simulink model "MiniHR"  (R2023a)
settings: Solver=FixedStepAuto  StartTime=0.0  StopTime=90  RelTol=1e-3
PreLoadFcn:
  | k=0.0001;
InitFcn:
  | k=0.0001;
values from neighbouring files (symbols this model uses):
  X = T(4)    [arm_contr.m]
  Y = T(5)    [arm_contr.m]
  Z = T(6)    [arm_contr.m]
libraries: sm_lib x208, nesl_utility x28, simulink x2
(part 2 of 6)

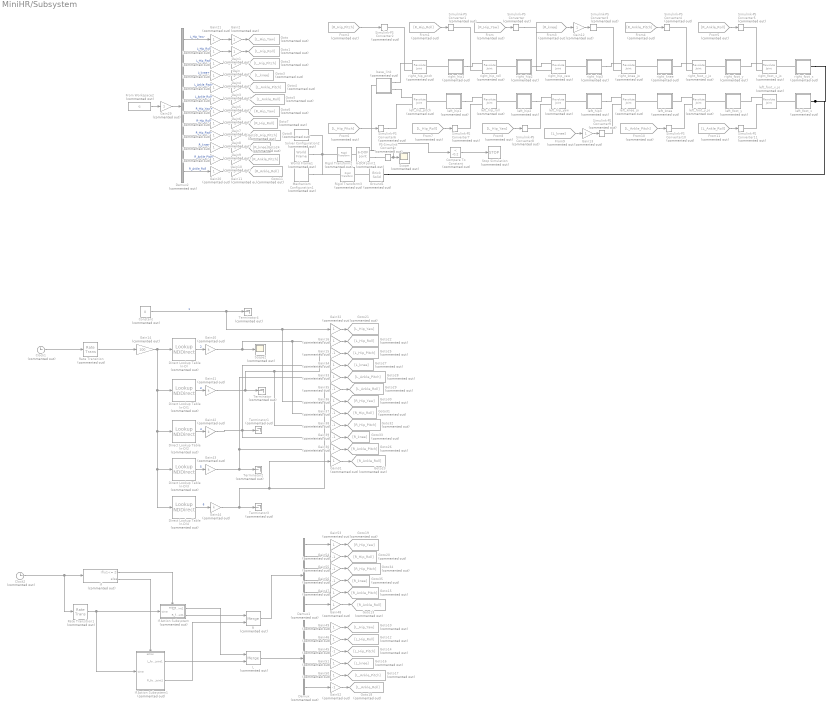
== system MiniHR/Subsystem ==
  6-DOF Joint1 : sm_lib/Joints/6-DOF Joint  Commented=on  JointMode=Normal  SenseConstraintForce=off  SenseConstraintForceX=off  SenseConstraintForceY=off  SenseConstraintForceZ=off  SenseConstraintTorque=off  SenseConstraintTorqueX=off  SenseConstraintTorqueY=off  SenseConstraintTorqueZ=off  SenseTotalForce=off  SenseTotalForceX=off  SenseTotalForceY=off  SenseTotalForceZ=off  SenseTotalTorque=off  SenseTotalTorqueX=off  SenseTotalTorqueY=off  SenseTotalTorqueZ=off  CompositeWrenchDir=FollowerOnBase  CompositeWrenchFrame=BaseFrame  PxEquilibriumPosition=0  PxEquilibriumPositionUnits=m  PxSpringStiffness=0  PxSpringStiffnessUnits=N/m  PxDampingCoefficient=0  PxDampingCoefficientUnits=N/(m/s)  PxTorqueActuationMode=NoTorque  PxMotionActuationMode=ComputedMotion  PxSensePosition=off  PxSenseVelocity=off  PxSenseAcceleration=off  PxSenseTorqueForce=off  PxSenseLowerLimitTorqueForce=off  PxSenseUpperLimitTorqueForce=off  PxLowerLimitSpecify=off  PxLowerLimitBound=-1  PxLowerLimitBoundUnits=m  PxLowerLimitStiffness=1e6  PxLowerLimitStiffnessUnits=N/m  PxLowerLimitDamping=1e3  PxLowerLimitDampingUnits=N/(m/s)  PxLowerLimitTransitionRegionWidth=1e-4  PxLowerLimitTransitionRegionWidthUnits=m  PxUpperLimitSpecify=off  PxUpperLimitBound=1  PxUpperLimitBoundUnits=m  PxUpperLimitStiffness=1e6  PxUpperLimitStiffnessUnits=N/m  PxUpperLimitDamping=1e3  PxUpperLimitDampingUnits=N/(m/s)  PxUpperLimitTransitionRegionWidth=1e-4  PxUpperLimitTransitionRegionWidthUnits=m  PxPositionTargetSpecify=off  PxPositionTargetPriority=High  PxPositionTargetValue=0  PxPositionTargetValueUnits=m  PxVelocityTargetSpecify=off  PxVelocityTargetPriority=High  PxVelocityTargetValue=0  PxVelocityTargetValueUnits=m/s  PyEquilibriumPosition=0  PyEquilibriumPositionUnits=m  PySpringStiffness=0  PySpringStiffnessUnits=N/m  PyDampingCoefficient=0  PyDampingCoefficientUnits=N/(m/s)  PyTorqueActuationMode=NoTorque  PyMotionActuationMode=ComputedMotion  PySensePosition=off  PySenseVelocity=off  PySenseAcceleration=off  PySenseTorqueForce=off  PySenseLowerLimitTorqueForce=off  PySenseUpperLimitTorqueForce=off  PyLowerLimitSpecify=off  PyLowerLimitBound=-1  PyLowerLimitBoundUnits=m  PyLowerLimitStiffness=1e6  PyLowerLimitStiffnessUnits=N/m  PyLowerLimitDamping=1e3  PyLowerLimitDampingUnits=N/(m/s)  PyLowerLimitTransitionRegionWidth=1e-4  PyLowerLimitTransitionRegionWidthUnits=m  PyUpperLimitSpecify=off  PyUpperLimitBound=1  PyUpperLimitBoundUnits=m  PyUpperLimitStiffness=1e6  PyUpperLimitStiffnessUnits=N/m  PyUpperLimitDamping=1e3  PyUpperLimitDampingUnits=N/(m/s)  PyUpperLimitTransitionRegionWidth=1e-4  PyUpperLimitTransitionRegionWidthUnits=m  PyPositionTargetSpecify=off  PyPositionTargetPriority=High  PyPositionTargetValue=0  PyPositionTargetValueUnits=m  PyVelocityTargetSpecify=off  PyVelocityTargetPriority=High  PyVelocityTargetValue=0  PyVelocityTargetValueUnits=m/s  PzEquilibriumPosition=0  PzEquilibriumPositionUnits=m  PzSpringStiffness=0  PzSpringStiffnessUnits=N/m  PzDampingCoefficient=0  PzDampingCoefficientUnits=N/(m/s)  PzTorqueActuationMode=NoTorque  PzMotionActuationMode=ComputedMotion  PzSensePosition=on  PzSenseVelocity=off  PzSenseAcceleration=off  PzSenseTorqueForce=off  PzSenseLowerLimitTorqueForce=off  PzSenseUpperLimitTorqueForce=off  PzLowerLimitSpecify=off  PzLowerLimitBound=-1  PzLowerLimitBoundUnits=m  PzLowerLimitStiffness=1e6  PzLowerLimitStiffnessUnits=N/m  PzLowerLimitDamping=1e3  PzLowerLimitDampingUnits=N/(m/s)  PzLowerLimitTransitionRegionWidth=1e-4  PzLowerLimitTransitionRegionWidthUnits=m  PzUpperLimitSpecify=off  PzUpperLimitBound=1  PzUpperLimitBoundUnits=m  PzUpperLimitStiffness=1e6  PzUpperLimitStiffnessUnits=N/m  PzUpperLimitDamping=1e3  PzUpperLimitDampingUnits=N/(m/s)  PzUpperLimitTransitionRegionWidth=1e-4  PzUpperLimitTransitionRegionWidthUnits=m  PzPositionTargetSpecify=off  PzPositionTargetPriority=High  PzPositionTargetValue=0  PzPositionTargetValueUnits=m  PzVelocityTargetSpecify=off  PzVelocityTargetPriority=High  PzVelocityTargetValue=0  PzVelocityTargetValueUnits=m/s  SphEqPosRotationMethod=None  SphEqPosRotationAngleUnits=deg  SphEqPosRotationStandardAxis=+Z  SphEqPosRotationAngle=0.0  SphEqPosRotationArbitraryAxis=[0 0 1]  SphEqPosFollAlignAxisA=+X  SphEqPosBaseAlignAxisA=+Y  SphEqPosFollAlignAxisB=+Y  SphEqPosBaseAlignAxisB=+Z  SphEqPosRotationSequenceAxes=FollowerAxes  SphEqPosRotationSequence=XYX  SphEqPosRotationSequenceAngles=[0 0 0]  SphEqPosRotationSequenceAnglesUnits=deg  SphEqPosRotationMatrix=[1 0 0; 0 1 0; 0 0 1]  SphEqPosQuaternion=[1 0 0 0]  SphSpringStiffness=0  SphSpringStiffnessUnits=N*m/deg  SphDampingCoefficient=0  SphDampingCoefficientUnits=N*m/(deg/s)  SphActuateTorqueX=off  SphActuateTorqueY=off  SphActuateTorqueZ=off  SphActuateTorque=off  SphTorqueActuationMode=NoTorque  SphMotionActuationMode=ComputedMotion  SphActuationFrame=BaseFrame  SphSensePosition=off  SphSenseVelocityX=off  SphSenseVelocityY=off  SphSenseVelocityZ=off  SphSenseVelocity=off  SphSenseAccelerationX=off  SphSenseAccelerationY=off  SphSenseAccelerationZ=off  SphSenseAcceleration=off  SphSenseTorqueX=off  SphSenseTorqueY=off  SphSenseTorqueZ=off  SphSenseTorqueForce=off  SphSenseLowerLimitTorqueMag=off  SphSenseUpperLimitTorqueMag=off  SphSensingFrame=BaseFrame  SphLowerLimitSpecify=off  SphLowerLimitBound=15  SphLowerLimitBoundUnits=deg  SphLowerLimitStiffness=1e4  SphLowerLimitStiffnessUnits=N*m/deg  SphLowerLimitDamping=10  SphLowerLimitDampingUnits=N*m/(deg/s)  SphLowerLimitTransitionRegionWidth=0.1  SphLowerLimitTransitionRegionWidthUnits=deg  SphUpperLimitSpecify=off  SphUpperLimitBound=45  SphUpperLimitBoundUnits=deg  SphUpperLimitStiffness=1e4  SphUpperLimitStiffnessUnits=N*m/deg  SphUpperLimitDamping=10  SphUpperLimitDampingUnits=N*m/(deg/s)  SphUpperLimitTransitionRegionWidth=0.1  SphUpperLimitTransitionRegionWidthUnits=deg  SphPositionTargetRotationMethod=None  SphPositionTargetRotationAngleUnits=deg  SphPositionTargetRotationStandardAxis=+Z  SphPositionTargetRotationAngle=0.0  SphPositionTargetRotationArbitraryAxis=[0 0 1]  SphPositionTargetFollAlignAxisA=+X  SphPositionTargetBaseAlignAxisA=+Y  SphPositionTargetFollAlignAxisB=+Y  SphPositionTargetBaseAlignAxisB=+Z  SphPositionTargetRotationSequenceAxes=FollowerAxes  SphPositionTargetRotationSequence=XYX  SphPositionTargetRotationSequenceAngles=[0 0 0]  SphPositionTargetRotationSequenceAnglesUnits=deg  SphPositionTargetRotationMatrix=[1 0 0; 0 1 0; 0 0 1]  SphPositionTargetQuaternion=[1 0 0 0]  SphPositionTargetSpecify=off  SphPositionTargetPriority=High  SphVelocityTargetValue=[0 0 0]  SphVelocityTargetValueUnits=deg/s  SphVelocityTargetSpecify=off  SphVelocityTargetPriority=High  SphVelocityTargetInFollowerFrame=on
  Clock1 : Clock  Commented=on
  Clock2 : Clock  Commented=on
      settings: Decimation=5
  Compare To Constant : simulink/Logic and Bit Operations/Compare To Constant  Commented=on  relop=<  const=-0.2  OutDataTypeStr=boolean
  Constant : Constant  Commented=on  Value=0  SampleTime=0.01
  Demux : Demux  Commented=on  Outputs=6
  Demux1 : Demux  Commented=on  Outputs=6
  Demux2 : Demux  Commented=on  Outputs=12
  Direct Lookup Table (n-D) : LookupNDDirect  Commented=on  NumberOfTableDimensions=1  Table=[0;0;0;0;0;0;0;0;0;0;0;0;0;0;0;0;0;0;0;0;0;0;0;0;0;0;0;0;0;0;0;0;0;0;0;0;0;0;0;0;0;0;0;0;0;0;0;0;0;0;0;0;0;0;0;0;0;0;0;0;0;0;0;0;0;0;0;0;0;0;0;0;0;0;0;0;0;0;0;0;0;0;0;0;0;0;0;0;0;0;0;0;0;0;0;0;0;0;0;0;0;0;0;0;0;-1;-1;-2;-4;-6;-9;-12;-17;-22;-29;-37;-46;-57;-69;-83;-99;-117;-137;-159;-183;-209;-238;-269;-303;-339;-378;-420;-463;-510;-559;-610;-664;-720;-779;-839;-902;-966;-1032;-1100;-1169;-1238;-1309;-1380;-1451;-1523;-1593;-1664;-1733;-1802;-1873;-1945;-2018;-2091;-2165;-2238;-2311;-2382;-2452;-2519;-2584;-2644;-2700;-2751;-2795;-2832;-2861;-2882;-2892;-2892;-2881;-2857;-2824;-2781;-2725;-2658;-2580;-2493;-2397;-2294;-2183;-2067;-1946;-1821;-1693;-1562;-1428;-1293;-1157;-1020;-882;-744;-605;-466;-327;-187;-47]  RemoveProtectionInput=on
  Direct Lookup Table (n-D)1 : LookupNDDirect  Commented=on  NumberOfTableDimensions=1  Table=[0;0;0;0;0;0;0;0;0;0;0;0;0;0;0;0;0;0;0;0;0;0;0;0;0;0;0;0;0;0;0;0;0;0;0;0;0;0;0;0;0;0;0;0;0;0;0;0;0;0;223;277;396;536;683;832;981;1128;1274;1418;1560;1699;1837;1971;2103;2233;2360;2484;2606;2724;2840;2953;3063;3170;3273;3374;3472;3566;3657;3745;3830;3911;3989;4063;4134;4201;4264;4324;4380;4432;4480;4524;4564;4600;4631;4658;4681;4698;4711;4719;4719;4719;4719;4719;4719;4719;4719;4719;4719;4719;4719;4719;4719;4719;4719;4719;4719;4719;4719;4719;4718;4718;4718;4717;4717;4716;4716;4715;4713;4712;4710;4708;4706;4703;4700;4696;4692;4687;4682;4676;4669;4662;4654;4645;4635;4624;4613;4601;4588;4574;4560;4545;4530;4524;4538;4568;4614;4671;4739;4816;4898;4984;5072;5161;5249;5335;5418;5495;5567;5633;5692;5742;5783;5815;5835;5845;5848;5846;5830;5803;5766;5719;5663;5599;5529;5452;5372;5287;5201;5114;5029;4946;4869;4799;4738;4689;4655;4637;4638;4648;4655]  RemoveProtectionInput=on
  Direct Lookup Table (n-D)2 : LookupNDDirect  Commented=on  NumberOfTableDimensions=1  Table=[0;0;0;0;0;0;0;0;0;0;0;0;0;0;0;0;0;0;0;0;0;0;0;0;0;0;0;0;0;0;0;0;0;0;0;0;0;0;0;0;0;0;0;0;0;0;0;0;0;0;552;688;983;1332;1697;2067;2437;2805;3169;3528;3883;4233;4578;4917;5250;5577;5899;6214;6523;6826;7123;7412;7695;7972;8241;8503;8758;9005;9244;9476;9700;9916;10123;10322;10511;10692;10864;11026;11178;11320;11452;11573;11683;11781;11868;11943;12005;12054;12090;12112;12112;12112;12112;12112;12112;12112;12112;12112;12112;12112;12112;12112;12112;12112;12112;12112;12112;12112;12111;12111;12110;12110;12109;12108;12106;12105;12103;12100;12097;12093;12088;12082;12076;12068;12059;12049;12037;12024;12009;11992;11974;11953;11930;11905;11878;11849;11817;11784;11748;11711;11671;11631;11588;11573;11611;11694;11819;11980;12169;12382;12614;12858;13110;13366;13622;13873;14117;14349;14566;14766;14944;15100;15228;15326;15392;15420;15432;15424;15376;15291;15174;15028;14856;14662;14449;14221;13981;13733;13482;13231;12986;12751;12532;12335;12165;12029;11933;11884;11887;11914;11934]  RemoveProtectionInput=on
  Direct Lookup Table (n-D)3 : LookupNDDirect  Commented=on  NumberOfTableDimensions=1  Table=[0;0;0;0;0;0;0;0;0;0;0;0;0;0;0;0;0;0;0;0;0;0;0;0;0;0;0;0;0;0;0;0;0;0;0;0;0;0;0;0;0;0;0;0;0;0;0;0;0;0;330;411;587;795;1014;1235;1456;1676;1895;2110;2323;2534;2741;2945;3146;3344;3539;3730;3918;4102;4283;4460;4633;4802;4967;5129;5286;5439;5587;5731;5870;6005;6134;6259;6378;6491;6599;6702;6798;6888;6972;7048;7119;7181;7237;7285;7324;7356;7379;7393;7393;7393;7393;7393;7393;7393;7393;7393;7393;7393;7393;7393;7393;7393;7393;7393;7393;7393;7393;7392;7392;7392;7391;7390;7389;7388;7387;7385;7383;7381;7378;7374;7370;7365;7359;7353;7345;7337;7327;7316;7304;7291;7277;7261;7243;7225;7204;7183;7160;7136;7111;7085;7059;7049;7073;7126;7206;7308;7430;7567;7716;7874;8038;8205;8373;8538;8699;8853;8998;9132;9253;9358;9445;9512;9556;9576;9584;9578;9545;9488;9408;9309;9193;9063;8920;8768;8609;8446;8281;8117;7957;7805;7663;7536;7427;7340;7278;7247;7249;7266;7279]  RemoveProtectionInput=on
  Direct Lookup Table (n-D)4 : LookupNDDirect  Commented=on  NumberOfTableDimensions=1  Table=[0;0;0;0;0;0;0;0;0;0;0;0;0;0;0;0;0;0;0;0;0;0;0;0;0;0;0;0;0;0;0;0;0;0;0;0;0;0;0;0;0;0;0;0;0;0;0;0;0;0;0;0;0;0;0;0;0;0;0;0;0;0;0;0;0;0;0;0;0;0;0;0;0;0;0;0;0;0;0;0;0;0;0;0;0;0;0;0;0;0;0;0;0;0;0;0;0;0;0;0;0;0;0;0;0;1;1;2;4;6;9;12;17;22;29;37;46;57;69;83;99;117;137;159;183;209;238;269;303;339;378;420;463;510;559;610;664;720;779;839;902;966;1032;1100;1169;1238;1309;1380;1451;1523;1593;1664;1733;1802;1873;1945;2018;2091;2165;2238;2311;2382;2452;2519;2584;2644;2700;2751;2795;2832;2861;2882;2892;2892;2881;2857;2824;2781;2725;2658;2580;2493;2397;2294;2183;2067;1946;1821;1693;1562;1428;1293;1157;1020;882;744;605;466;327;187;47]  RemoveProtectionInput=on
  From : From  Commented=on  GotoTag=R_Hip_Yaw
  From Workspace2 : FromWorkspace  Commented=on  VariableName=q
  From1 : From  Commented=on  GotoTag=R_Hip_Roll
  From10 : From  Commented=on  GotoTag=L_Ankle_Pitch
  From11 : From  Commented=on  GotoTag=L_Ankle_Roll
  From2 : From  Commented=on  GotoTag=R_Hip_Pitch
  From3 : From  Commented=on  GotoTag=R_knee
  From4 : From  Commented=on  GotoTag=R_Ankle_Pitch
  From5 : From  Commented=on  GotoTag=R_Ankle_Roll
  From6 : From  Commented=on  GotoTag=L_Hip_Pitch
  From7 : From  Commented=on  GotoTag=L_Hip_Roll
  From8 : From  Commented=on  GotoTag=L_Hip_Yaw
  From9 : From  Commented=on  GotoTag=L_knee
  Gain{,5,7..9,15,35,37..39,45,52,54..56} (15 alike) : Gain  Commented=on  Gain=-1
  Gain{1..4,6,10..13,16..34,36,46..51,53} (36 alike) : Gain  Commented=on
  Gain14 : Gain  Commented=on  Gain=100
  Gain{40..44} (5 alike) : Gain  Commented=on  Gain=k
  Goto : Goto  Commented=on  GotoTag=L_Hip_Yaw
  Goto1 : Goto  Commented=on  GotoTag=L_Hip_Roll
  Goto10 : Goto  Commented=on  GotoTag=L_Hip_Yaw
  Goto11 : Goto  Commented=on  GotoTag=R_Ankle_Roll
  Goto12 : Goto  Commented=on  GotoTag=L_Hip_Roll
  Goto13 : Goto  Commented=on  GotoTag=R_Ankle_Roll
  Goto14 : Goto  Commented=on  GotoTag=L_Hip_Pitch
  Goto15 : Goto  Commented=on  GotoTag=R_Ankle_Pitch
  Goto16 : Goto  Commented=on  GotoTag=L_knee
  Goto17 : Goto  Commented=on  GotoTag=L_Ankle_Pitch
  Goto18 : Goto  Commented=on  GotoTag=L_Ankle_Roll
  Goto19 : Goto  Commented=on  GotoTag=R_Hip_Yaw
  Goto2 : Goto  Commented=on  GotoTag=L_Hip_Pitch
  Goto20 : Goto  Commented=on  GotoTag=R_Hip_Roll
  Goto21 : Goto  Commented=on  GotoTag=L_Hip_Yaw
  Goto22 : Goto  Commented=on  GotoTag=L_Hip_Roll
  Goto23 : Goto  Commented=on  GotoTag=R_Ankle_Roll
  Goto24 : Goto  Commented=on  GotoTag=R_Ankle_Pitch
  Goto25 : Goto  Commented=on  GotoTag=L_Hip_Pitch
  Goto26 : Goto  Commented=on  GotoTag=R_Ankle_Pitch
  Goto27 : Goto  Commented=on  GotoTag=L_knee
  Goto28 : Goto  Commented=on  GotoTag=L_Ankle_Pitch
  Goto29 : Goto  Commented=on  GotoTag=L_Ankle_Roll
  Goto3 : Goto  Commented=on  GotoTag=L_knee
  Goto30 : Goto  Commented=on  GotoTag=R_Hip_Yaw
  Goto31 : Goto  Commented=on  GotoTag=R_Hip_Roll
  Goto32 : Goto  Commented=on  GotoTag=R_Hip_Pitch
  Goto33 : Goto  Commented=on  GotoTag=R_knee
  Goto34 : Goto  Commented=on  GotoTag=R_Hip_Pitch
  Goto35 : Goto  Commented=on  GotoTag=R_knee
  Goto4 : Goto  Commented=on  GotoTag=L_Ankle_Pitch
  Goto5 : Goto  Commented=on  GotoTag=L_Ankle_Roll
  Goto6 : Goto  Commented=on  GotoTag=R_Hip_Yaw
  Goto7 : Goto  Commented=on  GotoTag=R_Hip_Roll
  Goto8 : Goto  Commented=on  GotoTag=R_Hip_Pitch
  Goto9 : Goto  Commented=on  GotoTag=R_knee
  Ground1 : sm_lib/Body Elements/Brick Solid  Commented=on  GraphicAmbientColor=[0.15 0.15 0.15 1.0]  BasedOnType=Density  BrickDimensions=[10 10 0.1]  BrickDimensionsUnits=m  CenterOfMass=[0 0 0]  CenterOfMassUnits=m  GraphicDiffuseColor=[0.0 0.8 0.6]  Density=1000  DensityUnits=kg/m^3  DoExposeReferenceFrame=on  GraphicEmissiveColor=[0.0 0.0 0.0 1.0]  ExportEntireGeometry=on  SerializedFrames=<Frames/>  MarkerShape=Sphere  MarkerSize=10  GraphicType=FromGeometry  InertiaType=CalculateFromGeometry  Mass=1  MassUnits=kg  MomentsOfInertia=[1 1 1]  MomentsOfInertiaUnits=kg*m^2  GraphicOpacity=1.0  ProductsOfInertia=[0 0 0]  ProductsOfInertiaUnits=kg*m^2  GraphicShininess=75  GraphicSpecularColor=[0.5 0.5 0.5 1.0]  GraphicVisPropType=SimpleVisualProperties
  If : If  Commented=on  IfExpression=u1<= 2
  If Action Subsystem : Subsystem  Commented=on  TreatAsAtomicUnit=on
  If Action Subsystem1 : Subsystem  Commented=on  TreatAsAtomicUnit=on
  L : Merge  Commented=on
  Mechanism Configuration1 : sm_lib/Utilities/Mechanism Configuration  Commented=on  UniformGravity=Constant  GravityVector=[0 0 -9.80665]  GravityVectorUnits=m/s^2  LinearizationDelta=0.001  JointModeTransitionNonlinearIterations=2
  PS-Simulink Converter : nesl_utility/PS-Simulink Converter  Commented=on  PhysicalDomain=network_engine_domain  SubClassName=ps_output  LeftPortType=input  RightPortType=output  PseudoPeriodic=off  Frequencies=[]  VectorFormat=inherit  Unit=inherit  AffineConversion=off
  R : Merge  Commented=on
  Rate Transition : RateTransition  Commented=on  OutPortSampleTime=0.01
  Rate Transition1 : RateTransition  Commented=on  OutPortSampleTime=0.01
  Rigid Transform2 : sm_lib/Frames and Transforms/Rigid Transform  Commented=on  TranslationMethod=Cartesian  TranslationStandardOffset=0  TranslationStandardOffsetUnits=m  TranslationStandardAxis=+Z  TranslationCartesianOffset=[0 0 0.378]  TranslationCartesianOffsetUnits=m  TranslationROffset=0  TranslationROffsetUnits=m  TranslationZOffset=0  TranslationZOffsetUnits=m  TranslationThetaOffset=0  TranslationThetaOffsetUnits=deg  RotationMethod=None  RotationAngleUnits=deg  RotationStandardAxis=+Z  RotationAngle=0.0  RotationArbitraryAxis=[0 0 1]  FollAlignAxisA=+X  BaseAlignAxisA=+Y  FollAlignAxisB=+Y  BaseAlignAxisB=+Z  RotationSequenceAxes=FollowerAxes  RotationSequence=XYX  RotationSequenceAngles=[0 0 0]  RotationSequenceAnglesUnits=deg  RotationMatrix=[1 0 0; 0 1 0; 0 0 1]  Quaternion=[1 0 0 0]
  Rigid Transform3 : sm_lib/Frames and Transforms/Rigid Transform  Commented=on  TranslationMethod=Cartesian  TranslationStandardOffset=0  TranslationStandardOffsetUnits=m  TranslationStandardAxis=+Z  TranslationCartesianOffset=[4.5 0 -0.05]  TranslationCartesianOffsetUnits=m  TranslationROffset=0  TranslationROffsetUnits=m  TranslationZOffset=0  TranslationZOffsetUnits=m  TranslationThetaOffset=0  TranslationThetaOffsetUnits=deg  RotationMethod=None  RotationAngleUnits=deg  RotationStandardAxis=+Z  RotationAngle=0.0  RotationArbitraryAxis=[0 0 1]  FollAlignAxisA=+X  BaseAlignAxisA=+Y  FollAlignAxisB=+Y  BaseAlignAxisB=+Z  RotationSequenceAxes=FollowerAxes  RotationSequence=XYX  RotationSequenceAngles=[0 0 0]  RotationSequenceAnglesUnits=deg  RotationMatrix=[1 0 0; 0 1 0; 0 0 1]  Quaternion=[1 0 0 0]
  Scope : Scope  Commented=on
  Scope2 : Scope  Commented=on
  Simulink-PS Converter{,1..11} (12 alike) : nesl_utility/Simulink-PS Converter  Commented=on  PhysicalDomain=network_engine_domain  SubClassName=ps_input  LeftPortType=input  RightPortType=output  PseudoPeriodic=off  Frequencies=[]  NoiseDistribution=none  NoiseParameters=[]  Unit=1  AffineConversion=off  FilteringAndDerivatives=filter  SimscapeFilterOrder=2  InputFilterTimeConstant=0.001  UdotUserProvided=0
  Solver Configuration2 : nesl_utility/Solver Configuration  Commented=on  PhysicalDomain=network_engine_domain  SubClassName=solver  LeftPortType=input  RightPortType=generic  Tones=[]  Harmonics=[]  SimulateNoise=off  Profile=off  UseLocalSampling=off  EnableSwitchedLinearOptims=on  FrequencyDomain=off  UseCCode=off  RelTol=0.001  AbsTol=1e-06  MinStep=1e-09  ToWorkspace=off  RevertToSquareIcSolve=off  NumHomotopyIterations=100  PhasorMode=off  PhasorModeNumHarmonics=1  ConsistencySolver=NEWTON_FTOL  IndexReductionMethod=DerivativeReplacement  DoDC=off  ResidualTolerance=1e-09  ConsistencyTolSource=GLOBAL  ConsistencyAbsTol=0.001  ConsistencyRelTol=0.001  ConsistencyTolFactor=0.001  UseLocalSolver=off  LocalSolverChoice=NE_BACKWARD_EULER_ADVANCER  ResolveIndetEquations=on  FunctionEvalNumThread=1  LocalSolverSampleTime=0.001  DoFixedCost=off  MaxNonlinIter=3  MaxModeIter=2  ComputeImpulses=off  ImpulseIterations=2  LinearAlgebra=Sparse  LinearAlgebraNumThread=0  EquationFormulation=NE_TIME_EF  DelaysMemoryBudget=1024  AutomaticFiltering=on  FilteringTimeConstant=0.001  PartitionStorageMethod=AS_NEEDED  PartitionMemoryBudget=1024  PartitionMethod=FAST
  Stop Simulation : Stop  Commented=on
  Terminator{,1..4} (5 alike) : Terminator  Commented=on
  World Frame1 : sm_lib/Frames and Transforms/World Frame  Commented=on
  base_link : Subsystem  Commented=on
  left_foot_x : Subsystem  Commented=on
  left_foot_x_jo : sm_lib/Joints/Revolute Joint  Commented=on  JointMode=Normal  SenseConstraintForce=off  SenseConstraintForceX=off  SenseConstraintForceY=off  SenseConstraintForceZ=off  SenseConstraintTorque=off  SenseConstraintTorqueX=off  SenseConstraintTorqueY=off  SenseConstraintTorqueZ=off  SenseTotalForce=off  SenseTotalForceX=off  SenseTotalForceY=off  SenseTotalForceZ=off  SenseTotalTorque=off  SenseTotalTorqueX=off  SenseTotalTorqueY=off  SenseTotalTorqueZ=off  CompositeWrenchDir=FollowerOnBase  CompositeWrenchFrame=BaseFrame  EquilibriumPosition=0  EquilibriumPositionUnits=deg  SpringStiffness=0  SpringStiffnessUnits=N*m/deg  DampingCoefficient=1  DampingCoefficientUnits=kg*m^2/(rad*s)  TorqueActuationMode=ComputedTorque  MotionActuationMode=InputMotion  SensePosition=off  SenseVelocity=off  SenseAcceleration=off  SenseTorqueForce=off  SenseLowerLimitTorqueForce=off  SenseUpperLimitTorqueForce=off  LowerLimitSpecify=on  LowerLimitBound=-3  LowerLimitBoundUnits=rad  LowerLimitStiffness=1e4  LowerLimitStiffnessUnits=N*m/deg  LowerLimitDamping=10  LowerLimitDampingUnits=N*m/(deg/s)  LowerLimitTransitionRegionWidth=0.1  LowerLimitTransitionRegionWidthUnits=deg  UpperLimitSpecify=on  UpperLimitBound=3  UpperLimitBoundUnits=rad  UpperLimitStiffness=1e4  UpperLimitStiffnessUnits=N*m/deg  UpperLimitDamping=10  UpperLimitDampingUnits=N*m/(deg/s)  UpperLimitTransitionRegionWidth=0.1  UpperLimitTransitionRegionWidthUnits=deg  PositionTargetSpecify=off  PositionTargetPriority=High  PositionTargetValue=0  PositionTargetValueUnits=deg  VelocityTargetSpecify=off  VelocityTargetPriority=High  VelocityTargetValue=0  VelocityTargetValueUnits=deg/s
  left_foot_y : Subsystem  Commented=on
  left_foot_y_jo : sm_lib/Joints/Revolute Joint  Commented=on  JointMode=Normal  SenseConstraintForce=off  SenseConstraintForceX=off  SenseConstraintForceY=off  SenseConstraintForceZ=off  SenseConstraintTorque=off  SenseConstraintTorqueX=off  SenseConstraintTorqueY=off  SenseConstraintTorqueZ=off  SenseTotalForce=off  SenseTotalForceX=off  SenseTotalForceY=off  SenseTotalForceZ=off  SenseTotalTorque=off  SenseTotalTorqueX=off  SenseTotalTorqueY=off  SenseTotalTorqueZ=off  CompositeWrenchDir=FollowerOnBase  CompositeWrenchFrame=BaseFrame  EquilibriumPosition=0  EquilibriumPositionUnits=deg  SpringStiffness=0  SpringStiffnessUnits=N*m/deg  DampingCoefficient=1  DampingCoefficientUnits=kg*m^2/(rad*s)  TorqueActuationMode=ComputedTorque  MotionActuationMode=InputMotion  SensePosition=off  SenseVelocity=off  SenseAcceleration=off  SenseTorqueForce=off  SenseLowerLimitTorqueForce=off  SenseUpperLimitTorqueForce=off  LowerLimitSpecify=on  LowerLimitBound=-3  LowerLimitBoundUnits=rad  LowerLimitStiffness=1e4  LowerLimitStiffnessUnits=N*m/deg  LowerLimitDamping=10  LowerLimitDampingUnits=N*m/(deg/s)  LowerLimitTransitionRegionWidth=0.1  LowerLimitTransitionRegionWidthUnits=deg  UpperLimitSpecify=on  UpperLimitBound=3  UpperLimitBoundUnits=rad  UpperLimitStiffness=1e4  UpperLimitStiffnessUnits=N*m/deg  UpperLimitDamping=10  UpperLimitDampingUnits=N*m/(deg/s)  UpperLimitTransitionRegionWidth=0.1  UpperLimitTransitionRegionWidthUnits=deg  PositionTargetSpecify=off  PositionTargetPriority=High  PositionTargetValue=0  PositionTargetValueUnits=deg  VelocityTargetSpecify=off  VelocityTargetPriority=High  VelocityTargetValue=0  VelocityTargetValueUnits=deg/s
  left_hip1 : Subsystem  Commented=on
  left_hip2 : Subsystem  Commented=on
  left_hip3 : Subsystem  Commented=on
  left_hip_pitch : sm_lib/Joints/Revolute Joint  Commented=on  JointMode=Normal  SenseConstraintForce=off  SenseConstraintForceX=off  SenseConstraintForceY=off  SenseConstraintForceZ=off  SenseConstraintTorque=off  SenseConstraintTorqueX=off  SenseConstraintTorqueY=off  SenseConstraintTorqueZ=off  SenseTotalForce=off  SenseTotalForceX=off  SenseTotalForceY=off  SenseTotalForceZ=off  SenseTotalTorque=off  SenseTotalTorqueX=off  SenseTotalTorqueY=off  SenseTotalTorqueZ=off  CompositeWrenchDir=FollowerOnBase  CompositeWrenchFrame=BaseFrame  EquilibriumPosition=0  EquilibriumPositionUnits=deg  SpringStiffness=0  SpringStiffnessUnits=N*m/deg  DampingCoefficient=1  DampingCoefficientUnits=kg*m^2/(rad*s)  TorqueActuationMode=ComputedTorque  MotionActuationMode=InputMotion  SensePosition=off  SenseVelocity=off  SenseAcceleration=off  SenseTorqueForce=off  SenseLowerLimitTorqueForce=off  SenseUpperLimitTorqueForce=off  LowerLimitSpecify=on  LowerLimitBound=-3  LowerLimitBoundUnits=rad  LowerLimitStiffness=1e4  LowerLimitStiffnessUnits=N*m/deg  LowerLimitDamping=10  LowerLimitDampingUnits=N*m/(deg/s)  LowerLimitTransitionRegionWidth=0.1  LowerLimitTransitionRegionWidthUnits=deg  UpperLimitSpecify=on  UpperLimitBound=3  UpperLimitBoundUnits=rad  UpperLimitStiffness=1e4  UpperLimitStiffnessUnits=N*m/deg  UpperLimitDamping=10  UpperLimitDampingUnits=N*m/(deg/s)  UpperLimitTransitionRegionWidth=0.1  UpperLimitTransitionRegionWidthUnits=deg  PositionTargetSpecify=off  PositionTargetPriority=High  PositionTargetValue=0  PositionTargetValueUnits=deg  VelocityTargetSpecify=off  VelocityTargetPriority=High  VelocityTargetValue=0  VelocityTargetValueUnits=deg/s
  left_hip_roll : sm_lib/Joints/Revolute Joint  Commented=on  JointMode=Normal  SenseConstraintForce=off  SenseConstraintForceX=off  SenseConstraintForceY=off  SenseConstraintForceZ=off  SenseConstraintTorque=off  SenseConstraintTorqueX=off  SenseConstraintTorqueY=off  SenseConstraintTorqueZ=off  SenseTotalForce=off  SenseTotalForceX=off  SenseTotalForceY=off  SenseTotalForceZ=off  SenseTotalTorque=off  SenseTotalTorqueX=off  SenseTotalTorqueY=off  SenseTotalTorqueZ=off  CompositeWrenchDir=FollowerOnBase  CompositeWrenchFrame=BaseFrame  EquilibriumPosition=0  EquilibriumPositionUnits=deg  SpringStiffness=0  SpringStiffnessUnits=N*m/deg  DampingCoefficient=1  DampingCoefficientUnits=kg*m^2/(rad*s)  TorqueActuationMode=ComputedTorque  MotionActuationMode=InputMotion  SensePosition=off  SenseVelocity=off  SenseAcceleration=off  SenseTorqueForce=off  SenseLowerLimitTorqueForce=off  SenseUpperLimitTorqueForce=off  LowerLimitSpecify=on  LowerLimitBound=-3  LowerLimitBoundUnits=rad  LowerLimitStiffness=1e4  LowerLimitStiffnessUnits=N*m/deg  LowerLimitDamping=10  LowerLimitDampingUnits=N*m/(deg/s)  LowerLimitTransitionRegionWidth=0.1  LowerLimitTransitionRegionWidthUnits=deg  UpperLimitSpecify=on  UpperLimitBound=3  UpperLimitBoundUnits=rad  UpperLimitStiffness=1e4  UpperLimitStiffnessUnits=N*m/deg  UpperLimitDamping=10  UpperLimitDampingUnits=N*m/(deg/s)  UpperLimitTransitionRegionWidth=0.1  UpperLimitTransitionRegionWidthUnits=deg  PositionTargetSpecify=off  PositionTargetPriority=High  PositionTargetValue=0  PositionTargetValueUnits=deg  VelocityTargetSpecify=off  VelocityTargetPriority=High  VelocityTargetValue=0  VelocityTargetValueUnits=deg/s
  left_hip_yaw : sm_lib/Joints/Revolute Joint  Commented=on  JointMode=Normal  SenseConstraintForce=off  SenseConstraintForceX=off  SenseConstraintForceY=off  SenseConstraintForceZ=off  SenseConstraintTorque=off  SenseConstraintTorqueX=off  SenseConstraintTorqueY=off  SenseConstraintTorqueZ=off  SenseTotalForce=off  SenseTotalForceX=off  SenseTotalForceY=off  SenseTotalForceZ=off  SenseTotalTorque=off  SenseTotalTorqueX=off  SenseTotalTorqueY=off  SenseTotalTorqueZ=off  CompositeWrenchDir=FollowerOnBase  CompositeWrenchFrame=BaseFrame  EquilibriumPosition=0  EquilibriumPositionUnits=deg  SpringStiffness=0  SpringStiffnessUnits=N*m/deg  DampingCoefficient=1  DampingCoefficientUnits=kg*m^2/(rad*s)  TorqueActuationMode=ComputedTorque  MotionActuationMode=InputMotion  SensePosition=off  SenseVelocity=off  SenseAcceleration=off  SenseTorqueForce=off  SenseLowerLimitTorqueForce=off  SenseUpperLimitTorqueForce=off  LowerLimitSpecify=on  LowerLimitBound=-3  LowerLimitBoundUnits=rad  LowerLimitStiffness=1e4  LowerLimitStiffnessUnits=N*m/deg  LowerLimitDamping=10  LowerLimitDampingUnits=N*m/(deg/s)  LowerLimitTransitionRegionWidth=0.1  LowerLimitTransitionRegionWidthUnits=deg  UpperLimitSpecify=on  UpperLimitBound=3  UpperLimitBoundUnits=rad  UpperLimitStiffness=1e4  UpperLimitStiffnessUnits=N*m/deg  UpperLimitDamping=10  UpperLimitDampingUnits=N*m/(deg/s)  UpperLimitTransitionRegionWidth=0.1  UpperLimitTransitionRegionWidthUnits=deg  PositionTargetSpecify=off  PositionTargetPriority=High  PositionTargetValue=0  PositionTargetValueUnits=deg  VelocityTargetSpecify=off  VelocityTargetPriority=High  VelocityTargetValue=0  VelocityTargetValueUnits=deg/s
  left_knee : Subsystem  Commented=on
  left_knee_jo : sm_lib/Joints/Revolute Joint  Commented=on  JointMode=Normal  SenseConstraintForce=off  SenseConstraintForceX=off  SenseConstraintForceY=off  SenseConstraintForceZ=off  SenseConstraintTorque=off  SenseConstraintTorqueX=off  SenseConstraintTorqueY=off  SenseConstraintTorqueZ=off  SenseTotalForce=off  SenseTotalForceX=off  SenseTotalForceY=off  SenseTotalForceZ=off  SenseTotalTorque=off  SenseTotalTorqueX=off  SenseTotalTorqueY=off  SenseTotalTorqueZ=off  CompositeWrenchDir=FollowerOnBase  CompositeWrenchFrame=BaseFrame  EquilibriumPosition=0  EquilibriumPositionUnits=deg  SpringStiffness=0  SpringStiffnessUnits=N*m/deg  DampingCoefficient=1  DampingCoefficientUnits=kg*m^2/(rad*s)  TorqueActuationMode=ComputedTorque  MotionActuationMode=InputMotion  SensePosition=off  SenseVelocity=off  SenseAcceleration=off  SenseTorqueForce=off  SenseLowerLimitTorqueForce=off  SenseUpperLimitTorqueForce=off  LowerLimitSpecify=on  LowerLimitBound=-3  LowerLimitBoundUnits=rad  LowerLimitStiffness=1e4  LowerLimitStiffnessUnits=N*m/deg  LowerLimitDamping=10  LowerLimitDampingUnits=N*m/(deg/s)  LowerLimitTransitionRegionWidth=0.1  LowerLimitTransitionRegionWidthUnits=deg  UpperLimitSpecify=on  UpperLimitBound=3  UpperLimitBoundUnits=rad  UpperLimitStiffness=1e4  UpperLimitStiffnessUnits=N*m/deg  UpperLimitDamping=10  UpperLimitDampingUnits=N*m/(deg/s)  UpperLimitTransitionRegionWidth=0.1  UpperLimitTransitionRegionWidthUnits=deg  PositionTargetSpecify=off  PositionTargetPriority=High  PositionTargetValue=0  PositionTargetValueUnits=deg  VelocityTargetSpecify=off  VelocityTargetPriority=High  VelocityTargetValue=0  VelocityTargetValueUnits=deg/s
  right_foot_x : Subsystem  Commented=on
  right_foot_x_jo : sm_lib/Joints/Revolute Joint  Commented=on  JointMode=Normal  SenseConstraintForce=off  SenseConstraintForceX=off  SenseConstraintForceY=off  SenseConstraintForceZ=off  SenseConstraintTorque=off  SenseConstraintTorqueX=off  SenseConstraintTorqueY=off  SenseConstraintTorqueZ=off  SenseTotalForce=off  SenseTotalForceX=off  SenseTotalForceY=off  SenseTotalForceZ=off  SenseTotalTorque=off  SenseTotalTorqueX=off  SenseTotalTorqueY=off  SenseTotalTorqueZ=off  CompositeWrenchDir=FollowerOnBase  CompositeWrenchFrame=BaseFrame  EquilibriumPosition=0  EquilibriumPositionUnits=deg  SpringStiffness=0  SpringStiffnessUnits=N*m/deg  DampingCoefficient=1  DampingCoefficientUnits=kg*m^2/(rad*s)  TorqueActuationMode=ComputedTorque  MotionActuationMode=InputMotion  SensePosition=off  SenseVelocity=off  SenseAcceleration=off  SenseTorqueForce=off  SenseLowerLimitTorqueForce=off  SenseUpperLimitTorqueForce=off  LowerLimitSpecify=on  LowerLimitBound=-3  LowerLimitBoundUnits=rad  LowerLimitStiffness=1e4  LowerLimitStiffnessUnits=N*m/deg  LowerLimitDamping=10  LowerLimitDampingUnits=N*m/(deg/s)  LowerLimitTransitionRegionWidth=0.1  LowerLimitTransitionRegionWidthUnits=deg  UpperLimitSpecify=on  UpperLimitBound=3  UpperLimitBoundUnits=rad  UpperLimitStiffness=1e4  UpperLimitStiffnessUnits=N*m/deg  UpperLimitDamping=10  UpperLimitDampingUnits=N*m/(deg/s)  UpperLimitTransitionRegionWidth=0.1  UpperLimitTransitionRegionWidthUnits=deg  PositionTargetSpecify=off  PositionTargetPriority=High  PositionTargetValue=0  PositionTargetValueUnits=deg  VelocityTargetSpecify=off  VelocityTargetPriority=High  VelocityTargetValue=0  VelocityTargetValueUnits=deg/s
  right_foot_y : Subsystem  Commented=on
  right_foot_y_jo : sm_lib/Joints/Revolute Joint  Commented=on  JointMode=Normal  SenseConstraintForce=off  SenseConstraintForceX=off  SenseConstraintForceY=off  SenseConstraintForceZ=off  SenseConstraintTorque=off  SenseConstraintTorqueX=off  SenseConstraintTorqueY=off  SenseConstraintTorqueZ=off  SenseTotalForce=off  SenseTotalForceX=off  SenseTotalForceY=off  SenseTotalForceZ=off  SenseTotalTorque=off  SenseTotalTorqueX=off  SenseTotalTorqueY=off  SenseTotalTorqueZ=off  CompositeWrenchDir=FollowerOnBase  CompositeWrenchFrame=BaseFrame  EquilibriumPosition=0  EquilibriumPositionUnits=deg  SpringStiffness=0  SpringStiffnessUnits=N*m/deg  DampingCoefficient=1  DampingCoefficientUnits=kg*m^2/(rad*s)  TorqueActuationMode=ComputedTorque  MotionActuationMode=InputMotion  SensePosition=off  SenseVelocity=off  SenseAcceleration=off  SenseTorqueForce=off  SenseLowerLimitTorqueForce=off  SenseUpperLimitTorqueForce=off  LowerLimitSpecify=on  LowerLimitBound=-3  LowerLimitBoundUnits=rad  LowerLimitStiffness=1e4  LowerLimitStiffnessUnits=N*m/deg  LowerLimitDamping=10  LowerLimitDampingUnits=N*m/(deg/s)  LowerLimitTransitionRegionWidth=0.1  LowerLimitTransitionRegionWidthUnits=deg  UpperLimitSpecify=on  UpperLimitBound=3  UpperLimitBoundUnits=rad  UpperLimitStiffness=1e4  UpperLimitStiffnessUnits=N*m/deg  UpperLimitDamping=10  UpperLimitDampingUnits=N*m/(deg/s)  UpperLimitTransitionRegionWidth=0.1  UpperLimitTransitionRegionWidthUnits=deg  PositionTargetSpecify=off  PositionTargetPriority=High  PositionTargetValue=0  PositionTargetValueUnits=deg  VelocityTargetSpecify=off  VelocityTargetPriority=High  VelocityTargetValue=0  VelocityTargetValueUnits=deg/s
  right_hip1 : Subsystem  Commented=on
  right_hip2 : Subsystem  Commented=on
  right_hip3 : Subsystem  Commented=on
  right_hip_pitch : sm_lib/Joints/Revolute Joint  Commented=on  JointMode=Normal  SenseConstraintForce=off  SenseConstraintForceX=off  SenseConstraintForceY=off  SenseConstraintForceZ=off  SenseConstraintTorque=off  SenseConstraintTorqueX=off  SenseConstraintTorqueY=off  SenseConstraintTorqueZ=off  SenseTotalForce=off  SenseTotalForceX=off  SenseTotalForceY=off  SenseTotalForceZ=off  SenseTotalTorque=off  SenseTotalTorqueX=off  SenseTotalTorqueY=off  SenseTotalTorqueZ=off  CompositeWrenchDir=FollowerOnBase  CompositeWrenchFrame=BaseFrame  EquilibriumPosition=0  EquilibriumPositionUnits=deg  SpringStiffness=0  SpringStiffnessUnits=N*m/deg  DampingCoefficient=1  DampingCoefficientUnits=kg*m^2/(rad*s)  TorqueActuationMode=ComputedTorque  MotionActuationMode=InputMotion  SensePosition=off  SenseVelocity=off  SenseAcceleration=off  SenseTorqueForce=off  SenseLowerLimitTorqueForce=off  SenseUpperLimitTorqueForce=off  LowerLimitSpecify=on  LowerLimitBound=-3  LowerLimitBoundUnits=rad  LowerLimitStiffness=1e4  LowerLimitStiffnessUnits=N*m/deg  LowerLimitDamping=10  LowerLimitDampingUnits=N*m/(deg/s)  LowerLimitTransitionRegionWidth=0.1  LowerLimitTransitionRegionWidthUnits=deg  UpperLimitSpecify=on  UpperLimitBound=3  UpperLimitBoundUnits=rad  UpperLimitStiffness=1e4  UpperLimitStiffnessUnits=N*m/deg  UpperLimitDamping=10  UpperLimitDampingUnits=N*m/(deg/s)  UpperLimitTransitionRegionWidth=0.1  UpperLimitTransitionRegionWidthUnits=deg  PositionTargetSpecify=off  PositionTargetPriority=High  PositionTargetValue=0  PositionTargetValueUnits=deg  VelocityTargetSpecify=off  VelocityTargetPriority=High  VelocityTargetValue=0  VelocityTargetValueUnits=deg/s
  right_hip_roll : sm_lib/Joints/Revolute Joint  Commented=on  JointMode=Normal  SenseConstraintForce=off  SenseConstraintForceX=off  SenseConstraintForceY=off  SenseConstraintForceZ=off  SenseConstraintTorque=off  SenseConstraintTorqueX=off  SenseConstraintTorqueY=off  SenseConstraintTorqueZ=off  SenseTotalForce=off  SenseTotalForceX=off  SenseTotalForceY=off  SenseTotalForceZ=off  SenseTotalTorque=off  SenseTotalTorqueX=off  SenseTotalTorqueY=off  SenseTotalTorqueZ=off  CompositeWrenchDir=FollowerOnBase  CompositeWrenchFrame=BaseFrame  EquilibriumPosition=0  EquilibriumPositionUnits=deg  SpringStiffness=0  SpringStiffnessUnits=N*m/deg  DampingCoefficient=1  DampingCoefficientUnits=kg*m^2/(rad*s)  TorqueActuationMode=ComputedTorque  MotionActuationMode=InputMotion  SensePosition=off  SenseVelocity=off  SenseAcceleration=off  SenseTorqueForce=off  SenseLowerLimitTorqueForce=off  SenseUpperLimitTorqueForce=off  LowerLimitSpecify=on  LowerLimitBound=-3  LowerLimitBoundUnits=rad  LowerLimitStiffness=1e4  LowerLimitStiffnessUnits=N*m/deg  LowerLimitDamping=10  LowerLimitDampingUnits=N*m/(deg/s)  LowerLimitTransitionRegionWidth=0.1  LowerLimitTransitionRegionWidthUnits=deg  UpperLimitSpecify=on  UpperLimitBound=3  UpperLimitBoundUnits=rad  UpperLimitStiffness=1e4  UpperLimitStiffnessUnits=N*m/deg  UpperLimitDamping=10  UpperLimitDampingUnits=N*m/(deg/s)  UpperLimitTransitionRegionWidth=0.1  UpperLimitTransitionRegionWidthUnits=deg  PositionTargetSpecify=off  PositionTargetPriority=High  PositionTargetValue=0  PositionTargetValueUnits=deg  VelocityTargetSpecify=off  VelocityTargetPriority=High  VelocityTargetValue=0  VelocityTargetValueUnits=deg/s
  right_hip_yaw : sm_lib/Joints/Revolute Joint  Commented=on  JointMode=Normal  SenseConstraintForce=off  SenseConstraintForceX=off  SenseConstraintForceY=off  SenseConstraintForceZ=off  SenseConstraintTorque=off  SenseConstraintTorqueX=off  SenseConstraintTorqueY=off  SenseConstraintTorqueZ=off  SenseTotalForce=off  SenseTotalForceX=off  SenseTotalForceY=off  SenseTotalForceZ=off  SenseTotalTorque=off  SenseTotalTorqueX=off  SenseTotalTorqueY=off  SenseTotalTorqueZ=off  CompositeWrenchDir=FollowerOnBase  CompositeWrenchFrame=BaseFrame  EquilibriumPosition=0  EquilibriumPositionUnits=deg  SpringStiffness=0  SpringStiffnessUnits=N*m/deg  DampingCoefficient=1  DampingCoefficientUnits=kg*m^2/(rad*s)  TorqueActuationMode=ComputedTorque  MotionActuationMode=InputMotion  SensePosition=off  SenseVelocity=off  SenseAcceleration=off  SenseTorqueForce=off  SenseLowerLimitTorqueForce=off  SenseUpperLimitTorqueForce=off  LowerLimitSpecify=on  LowerLimitBound=-3  LowerLimitBoundUnits=rad  LowerLimitStiffness=1e4  LowerLimitStiffnessUnits=N*m/deg  LowerLimitDamping=10  LowerLimitDampingUnits=N*m/(deg/s)  LowerLimitTransitionRegionWidth=0.1  LowerLimitTransitionRegionWidthUnits=deg  UpperLimitSpecify=on  UpperLimitBound=3  UpperLimitBoundUnits=rad  UpperLimitStiffness=1e4  UpperLimitStiffnessUnits=N*m/deg  UpperLimitDamping=10  UpperLimitDampingUnits=N*m/(deg/s)  UpperLimitTransitionRegionWidth=0.1  UpperLimitTransitionRegionWidthUnits=deg  PositionTargetSpecify=off  PositionTargetPriority=High  PositionTargetValue=0  PositionTargetValueUnits=deg  VelocityTargetSpecify=off  VelocityTargetPriority=High  VelocityTargetValue=0  VelocityTargetValueUnits=deg/s
  right_knee : Subsystem  Commented=on
  right_knee_jo : sm_lib/Joints/Revolute Joint  Commented=on  JointMode=Normal  SenseConstraintForce=off  SenseConstraintForceX=off  SenseConstraintForceY=off  SenseConstraintForceZ=off  SenseConstraintTorque=off  SenseConstraintTorqueX=off  SenseConstraintTorqueY=off  SenseConstraintTorqueZ=off  SenseTotalForce=off  SenseTotalForceX=off  SenseTotalForceY=off  SenseTotalForceZ=off  SenseTotalTorque=off  SenseTotalTorqueX=off  SenseTotalTorqueY=off  SenseTotalTorqueZ=off  CompositeWrenchDir=FollowerOnBase  CompositeWrenchFrame=BaseFrame  EquilibriumPosition=0  EquilibriumPositionUnits=deg  SpringStiffness=0  SpringStiffnessUnits=N*m/deg  DampingCoefficient=1  DampingCoefficientUnits=kg*m^2/(rad*s)  TorqueActuationMode=ComputedTorque  MotionActuationMode=InputMotion  SensePosition=off  SenseVelocity=off  SenseAcceleration=off  SenseTorqueForce=off  SenseLowerLimitTorqueForce=off  SenseUpperLimitTorqueForce=off  LowerLimitSpecify=on  LowerLimitBound=-3  LowerLimitBoundUnits=rad  LowerLimitStiffness=1e4  LowerLimitStiffnessUnits=N*m/deg  LowerLimitDamping=10  LowerLimitDampingUnits=N*m/(deg/s)  LowerLimitTransitionRegionWidth=0.1  LowerLimitTransitionRegionWidthUnits=deg  UpperLimitSpecify=on  UpperLimitBound=3  UpperLimitBoundUnits=rad  UpperLimitStiffness=1e4  UpperLimitStiffnessUnits=N*m/deg  UpperLimitDamping=10  UpperLimitDampingUnits=N*m/(deg/s)  UpperLimitTransitionRegionWidth=0.1  UpperLimitTransitionRegionWidthUnits=deg  PositionTargetSpecify=off  PositionTargetPriority=High  PositionTargetValue=0  PositionTargetValueUnits=deg  VelocityTargetSpecify=off  VelocityTargetPriority=High  VelocityTargetValue=0  VelocityTargetValueUnits=deg/s
  wires:
  Gain50/1 -> Goto17/1
  Gain49/1 -> Goto10/1
  If Action Subsystem/1(L_foot_joint1) -> L/1
  R/1 -> Demux1/1
  Gain36/1 -> Goto30/1
  Gain19/1 -> Gain10/1
  If Action Subsystem1/1(L_foot_joint1) -> L/2
  From5/1 -> Simulink-PS Converter5/1
  Clock2/1 -> Rate Transition1/1, If/1
  Gain38/1 -> Goto32/1
  Gain41/1 -> Gain38/1, Gain15/1, Terminator/1
  Gain42/1 -> Gain34/1, Gain39/1, Terminator1/1
  Gain13/1 -> Simulink-PS Converter9/1
  Gain18/1 -> Gain1/1
  From Workspace2/1 -> Gain29/1
  Gain16/1 -> Goto22/1
  Gain15/1 -> Goto25/1
  Gain37/1 -> Goto31/1
  Gain11/1 -> Goto11/1
  Direct Lookup Table (n-D)1/1 -> Gain41/1  "3"
  Gain14/1 -> Direct Lookup Table (n-D)1/1, Direct Lookup Table (n-D)2/1, Direct Lookup Table (n-D)3/1, Direct Lookup Table (n-D)4/1, Direct Lookup Table (n-D)/1
  From4/1 -> Simulink-PS Converter4/1
  From1/1 -> Simulink-PS Converter1/1
  Gain31/1 -> Goto23/1
  If/2 -> If Action Subsystem1/Action
  Constant/1 -> Gain36/1, Gain32/1, Terminator4/1  "1"
  Gain30/1 -> Goto26/1
  Gain20/1 -> Gain11/1
  L/1 -> Demux/1
  Gain/1 -> Goto2/1
  Gain24/1 -> Gain5/1
  Clock1/1 -> Rate Transition/1
  Gain22/1 -> Gain3/1
  Gain7/1 -> Goto7/1
  Gain25/1 -> Gain6/1
  If Action Subsystem1/2(R_foot_joint1) -> R/2
  Demux2/1 -> Gain21/1  "L_Hip_Yaw-"
  Demux2/12 -> Gain20/1  "R_Ankle_Roll"
  Gain4/1 -> Goto3/1
  Demux2/11 -> Gain19/1  "R_Ankle_Pitch-"
  Gain33/1 -> Goto28/1
  Demux2/7 -> Gain25/1  "R_Hip_Yaw+"
  Demux2/6 -> Gain24/1  "L_Ankle_Roll-"
  Demux2/4 -> Gain23/1  "L_knee+"
  Gain8/1 -> Goto8/1
  Gain12/1 -> Simulink-PS Converter3/1
  Rate Transition/1 -> Gain14/1
  From10/1 -> Simulink-PS Converter10/1
  From3/1 -> Gain12/1
  Gain6/1 -> Goto6/1
  Gain3/1 -> Goto4/1
  Gain2/1 -> Goto/1
  Gain1/1 -> Goto1/1
  From11/1 -> Simulink-PS Converter11/1
  From7/1 -> Simulink-PS Converter7/1
  Direct Lookup Table (n-D)2/1 -> Gain42/1  "4"
  From2/1 -> Simulink-PS Converter2/1
  Demux2/3 -> Gain17/1  "L_Hip_Pitch"
  From/1 -> Simulink-PS Converter/1
  Gain52/1 -> Goto18/1
  Demux/1 -> Gain49/1
  Gain47/1 -> Goto15/1
  Direct Lookup Table (n-D)3/1 -> Gain43/1  "5"
  Demux1/2 -> Gain54/1
  Demux1/4 -> Gain56/1
  Gain40/1 -> Gain37/1, Gain16/1, Scope2/1
  Gain29/1 -> Demux2/1
  Gain34/1 -> Goto27/1
  Demux2/9 -> Gain27/1  "R_Hip_Pitch-"
  Gain44/1 -> Gain31/1, Gain35/1, Terminator3/1
  From6/1 -> Simulink-PS Converter6/1
  Demux/5 -> Gain50/1
  Gain28/1 -> Gain9/1
  Demux1/1 -> Gain53/1
  Demux2/8 -> Gain26/1  "R_Hip_Roll-"
  Rate Transition1/1 -> If Action Subsystem1/1(time), If Action Subsystem/1(time)
  PS-Simulink Converter/1 -> Compare To Constant/1, Scope/1
  Demux2/2 -> Gain18/1  "L_Hip_Roll"
  Direct Lookup Table (n-D)/1 -> Gain40/1  "2"
  Gain35/1 -> Goto29/1
  Gain32/1 -> Goto21/1
  Demux/4 -> Gain51/1
  Gain43/1 -> Gain33/1, Gain30/1, Terminator2/1
  If/1 -> If Action Subsystem/Action
  Gain10/1 -> Goto24/1
  Demux/6 -> Gain52/1
  Demux2/5 -> Gain22/1  "L_Ankle_Pitch-"
  From9/1 -> Gain13/1
  Demux1/5 -> Gain47/1
  Demux/2 -> Gain46/1
  Gain54/1 -> Goto20/1
  Demux1/3 -> Gain55/1
  Gain46/1 -> Goto12/1
  Gain39/1 -> Goto33/1
  Gain9/1 -> Goto9/1
  Demux1/6 -> Gain48/1
  From8/1 -> Simulink-PS Converter8/1
  Gain21/1 -> Gain2/1
  Gain55/1 -> Goto34/1
  Demux2/10 -> Gain28/1  "R_knee-"
  Gain27/1 -> Gain8/1
  If Action Subsystem/2(R_foot_joint1) -> R/1
  Gain48/1 -> Goto13/1
  Gain23/1 -> Gain4/1
  Direct Lookup Table (n-D)4/1 -> Gain44/1  "6"
  Gain51/1 -> Goto16/1
  Gain56/1 -> Goto35/1
  Gain53/1 -> Goto19/1
  Gain17/1 -> Gain/1
  Compare To Constant/1 -> Stop Simulation/1
  Gain45/1 -> Goto14/1
  Gain5/1 -> Goto5/1
  Gain26/1 -> Gain7/1
  Demux/3 -> Gain45/1
  connections:
  Rigid Transform2/LConn1 -- World Frame1/RConn1 -- Mechanism Configuration1/RConn1 -- Rigid Transform3/LConn1 -- Solver Configuration2/RConn1
  left_foot_x/RConn1 -- right_foot_x/RConn1 -- Ground1/LConn1
  right_hip1/LConn1 -- right_hip_pitch/RConn1
  6-DOF Joint1/RConn1 -- base_link/LConn1
  left_hip1/RConn1 -- left_hip_roll/LConn1
  right_foot_x/LConn1 -- right_foot_x_jo/RConn1
  right_hip_pitch/LConn2 -- Simulink-PS Converter2/RConn1
  left_foot_y_jo/LConn2 -- Simulink-PS Converter10/RConn1
  Ground1/RConn1 -- Rigid Transform3/RConn1
  right_knee/LConn1 -- right_knee_jo/RConn1
  left_foot_x/LConn1 -- left_foot_x_jo/RConn1
  right_hip3/LConn1 -- right_hip_yaw/RConn1
  left_hip2/RConn1 -- left_hip_yaw/LConn1
  6-DOF Joint1/RConn2 -- PS-Simulink Converter/LConn1
  right_hip_roll/LConn2 -- Simulink-PS Converter1/RConn1
  right_foot_x_jo/LConn2 -- Simulink-PS Converter5/RConn1
  right_hip1/RConn1 -- right_hip_roll/LConn1
  right_hip3/RConn1 -- right_knee_jo/LConn1
  left_hip1/LConn1 -- left_hip_pitch/RConn1
  right_foot_y/LConn1 -- right_foot_y_jo/RConn1
  left_hip_yaw/LConn2 -- Simulink-PS Converter8/RConn1
  Rigid Transform2/RConn1 -- 6-DOF Joint1/LConn1
  left_hip3/RConn1 -- left_knee_jo/LConn1
  left_foot_x_jo/LConn1 -- left_foot_y/RConn1
  right_knee_jo/LConn2 -- Simulink-PS Converter3/RConn1
  left_foot_y_jo/LConn1 -- left_knee/RConn1
  left_knee_jo/LConn2 -- Simulink-PS Converter9/RConn1
  right_foot_x_jo/LConn1 -- right_foot_y/RConn1
  left_foot_y/LConn1 -- left_foot_y_jo/RConn1
  left_hip_roll/LConn2 -- Simulink-PS Converter7/RConn1
  base_link/RConn1 -- right_hip_pitch/LConn1
  right_foot_y_jo/LConn2 -- Simulink-PS Converter4/RConn1
  left_hip3/LConn1 -- left_hip_yaw/RConn1
  right_hip2/LConn1 -- right_hip_roll/RConn1
  right_foot_y_jo/LConn1 -- right_knee/RConn1
  left_knee/LConn1 -- left_knee_jo/RConn1
  Simulink-PS Converter/RConn1 -- right_hip_yaw/LConn2
  right_hip2/RConn1 -- right_hip_yaw/LConn1
  base_link/RConn2 -- left_hip_pitch/LConn1
  left_hip2/LConn1 -- left_hip_roll/RConn1
  left_foot_x_jo/LConn2 -- Simulink-PS Converter11/RConn1
  Simulink-PS Converter6/RConn1 -- left_hip_pitch/LConn2
